simulink model "High_pass_Filter"  (R2020b)
settings: Solver=VariableStepAuto  StartTime=0.0  StopTime=1  RelTol=1e-3
settings Model: Creator=153  LastModifiedBy=153

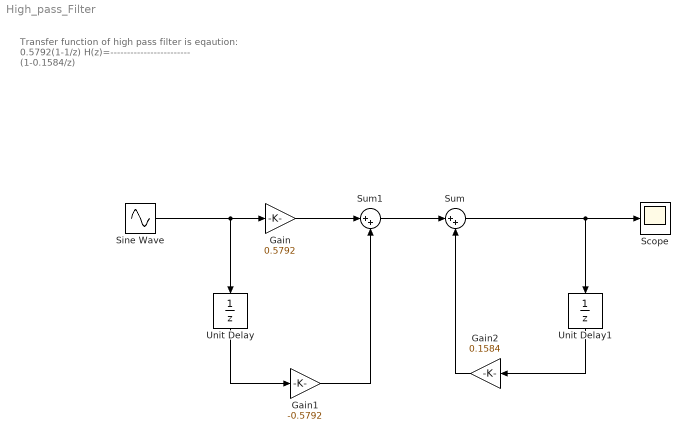
== system High_pass_Filter ==
  note: Transfer function of high pass filter is
      | eqaution:
      | 0.5792(1-1/z)
      | H(z)=------------------------
      | (1-0.1584/z)
  Gain : Gain  Gain=0.5792
  Gain1 : Gain  Gain=-0.5792
  Gain2 : Gain  Gain=0.1584
  Scope : Scope
  Sine Wave : Sin  Frequency=110  SampleTime=0
  Sum : Sum  Inputs=|++
  Sum1 : Sum  Inputs=|++
  Unit Delay : UnitDelay  SampleTime=-1  HasFrameUpgradeWarning=on
  Unit Delay1 : UnitDelay  SampleTime=-1  HasFrameUpgradeWarning=on
  wires:
  Sum/1 -> Unit Delay1/1, Scope/1
  Unit Delay1/1 -> Gain2/1
  Gain2/1 -> Sum/2
  Sine Wave/1 -> Unit Delay/1, Gain/1
  Unit Delay/1 -> Gain1/1
  Gain1/1 -> Sum1/2
  Gain/1 -> Sum1/1
  Sum1/1 -> Sum/1
